simulink model "White_Activity10_sim"  (R2020b)
settings: Solver=VariableStepAuto  StartTime=0.0  StopTime=5  RelTol=1e-3
settings Model: Creator=Michael  LastModifiedBy=Michael
settings OptimizationCC: BlockReduction=off  DefaultParameterBehavior=Inlined  BufferReuse=off

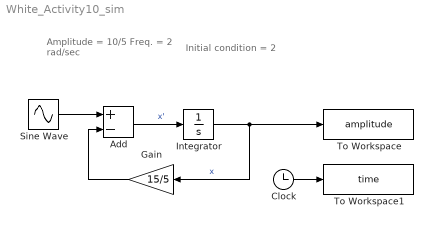
== system White_Activity10_sim ==
  note: Initial condition = 2
  note: Amplitude = 10/5
      | Freq. = 2 rad/sec
  Add : Sum  Inputs=+-
  Clock : Clock
  Gain : Gain  Gain=15/5
  Integrator : Integrator  InitialCondition=2
  Sine Wave : Sin  Amplitude=10/5  Frequency=2  SampleTime=0
  To Workspace : ToWorkspace  VariableName=amplitude  SampleTime=-1
  To Workspace1 : ToWorkspace  VariableName=time  SampleTime=-1
  wires:
  Sine Wave/1 -> Add/1
  Integrator/1 -> To Workspace/1, Gain/1  "x"
  Gain/1 -> Add/2
  Add/1 -> Integrator/1  "x'"
  Clock/1 -> To Workspace1/1
